simulink model "uavModel"  (R2023b)
settings: Solver=VariableStepAuto  StartTime=0.0  StopTime=10.0  RelTol=1e-3
InitFcn:
  | run('./config/config.m')
values from neighbouring files (symbols this model uses):
  mass = 11    [config_model.m]
undefined symbols (not defined in the file or in its folder): Cd, Cm, Earth, fractalcoef, lambda, propsMatrix, referenceHeight, WGS84, windSpeedInertial
libraries: aerolibasang x3, simulink_extras x1, aerolibtransform2 x1, aerolibatmos2 x1, shared6dof x1, sharedutil x1, sensorgpslib x1, mspsensorlib x1
settings Model: Creator=Rafael Blanco  LastModifiedBy=Victor

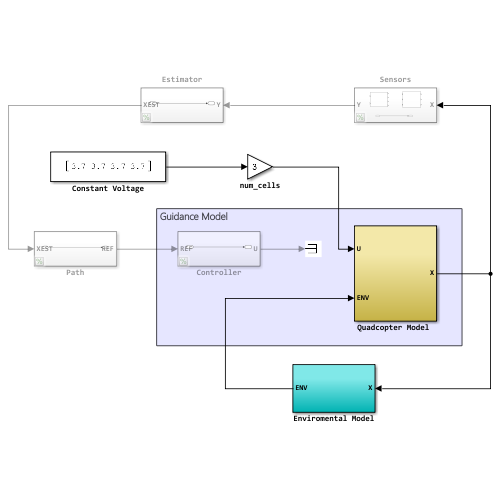
[thumbnail: Simulink's stored preview of the top-level diagram]
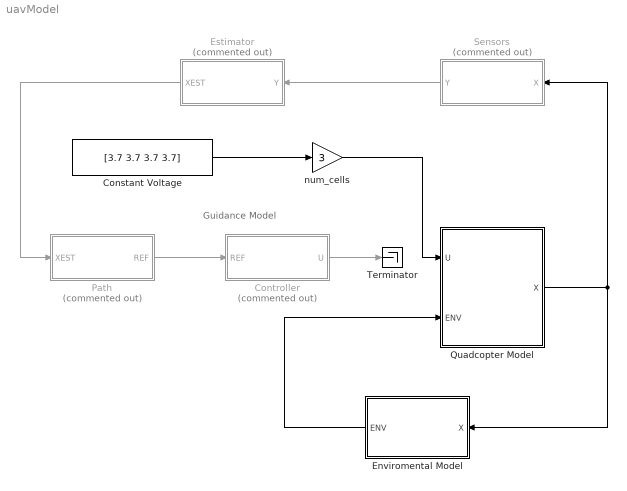
== system uavModel ==
  note: Guidance Model
  Constant Voltage : Constant  Value=[3.7 3.7 3.7 3.7]
  Controller : Subsystem  Commented=on
  Enviromental Model : Subsystem
  Estimator : Subsystem  Commented=on
  Path : Subsystem  Commented=on
  "Quadcopter Model " : Subsystem
  Sensors : Subsystem  Commented=on
  Terminator : Terminator
  num_cells : Gain  Gain=3
  wires:
  "Quadcopter Model "/1(X) -> Enviromental Model/1(X), Sensors/1(X)
  Enviromental Model/1(ENV) -> "Quadcopter Model "/2(ENV)
  Sensors/1(Y) -> Estimator/1(Y)
  Estimator/1(XEST) -> Path/1(XEST)
  Path/1(REF) -> Controller/1(REF)
  Controller/1(U) -> Terminator/1
  Constant Voltage/1 -> num_cells/1
  num_cells/1 -> "Quadcopter Model "/1(U)

== system uavModel/Controller ==
  REF : Inport
  U : Outport
  wires:
  REF/1 -> U/1

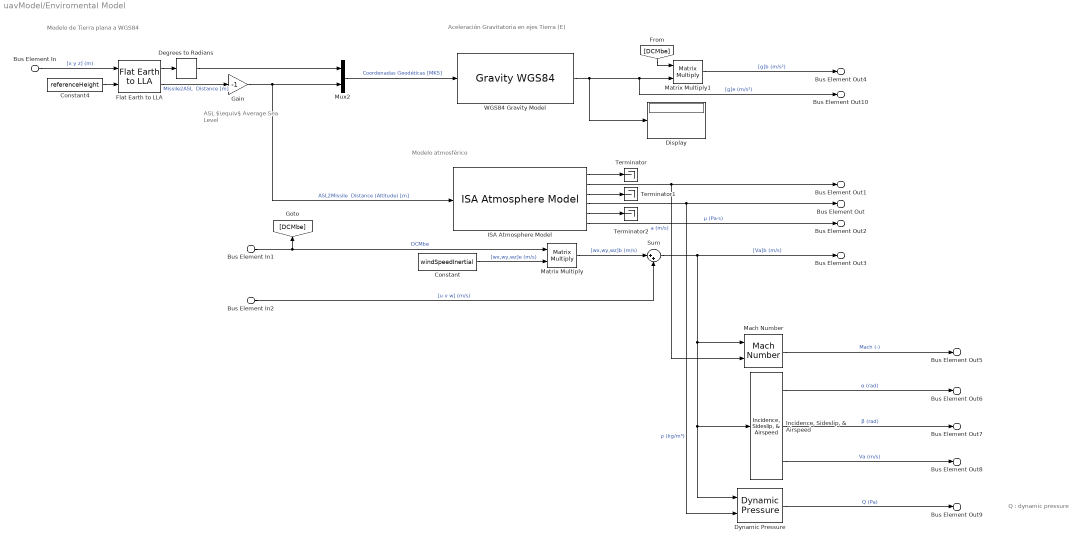
== system uavModel/Enviromental Model ==
  note: Modelo atmosférico
  note: Aceleración Gravitatoria en ejes Tierra (E)
  note: Modelo de Tierra plana a WGS84
  note: ASL $\equiv$ Average Sea Level
  note: Q : dynamic pressure
  Bus Element In2 : Inport  PortName=X  Element=[u v w] (m/s)
  Bus Element In : Inport  PortName=X  Element=[x y z] (m)
  Bus Element In1 : Inport  PortName=X  Element=DCMbe
  Constant : Constant  Value=windSpeedInertial
  Constant4 : Constant  Value=referenceHeight
  Degrees to Radians : simulink_extras/Transformations/Degrees to Radians
  Display : Display
  Dynamic Pressure : aerolibasang/Dynamic Pressure
  Flat Earth to LLA : aerolibtransform2/Flat Earth to LLA  units=Metric (MKS)  ptype=Earth (WGS84)  F=1/298.257223563  R=6378137  refPosPort=off  LL0=referenceGeodeticPosition  psi=0
  Gain : Gain  Gain=-1
  ISA Atmosphere Model : aerolibatmos2/ISA Atmosphere Model  useExtended=off  action=Warning  custom=off  viscosityOut=on  g=9.80665  gamma=1.4  R=287.0531  L=0.0065  h_trop=11000  h_strat=20000  rho0=1.225  P0=101325  T0=288.15  h0=0
  "Incidence, Sideslip, & Airspeed" : aerolibasang/Incidence, Sideslip, & Airspeed
  Mach Number : aerolibasang/Mach Number
  Matrix Multiply : Product  Multiplication=Matrix(*)
  Matrix Multiply1 : Product  Multiplication=Matrix(*)
  Mux2 : Mux  Inputs=2
  Sum : Sum  Inputs=|++
  Terminator : Terminator
  Terminator1 : Terminator
  Terminator2 : Terminator
  "WGS84 Gravity Model  " : GravityWGS84
  Bus Element Out : Outport  PortName=ENV  Element=ρ (kg/m³)
  Bus Element Out1 : Outport  PortName=ENV  Element=a (m/s)
  Bus Element Out2 : Outport  PortName=ENV  Element=μ (Pa·s)
  Bus Element Out3 : Outport  PortName=ENV  Element=[Va]b (m/s)
  Bus Element Out4 : Outport  PortName=ENV  Element=[g]b (m/s²)
  Bus Element Out5 : Outport  PortName=ENV  Element=Mach (-)
  Bus Element Out6 : Outport  PortName=ENV  Element=α (rad)
  Bus Element Out7 : Outport  PortName=ENV  Element=β (rad)
  Bus Element Out8 : Outport  PortName=ENV  Element=Va (m/s)
  Bus Element Out9 : Outport  PortName=ENV  Element=Q (Pa)
  Bus Element Out10 : Outport  PortName=ENV  Element=[g]e (m/s²)
  wires:
  "WGS84 Gravity Model  "/1 -> Bus Element Out10/1, Matrix Multiply1/2, Display/1  "[g]e (m/s²)"
  Mux2/1 -> "WGS84 Gravity Model  "/1  "Coordenadas Geodéticas [MKS]"
  Gain/1 -> Mux2/2, ISA Atmosphere Model/1  "ASL2Missile  Distance (Altitude) [m]"
  Flat Earth to LLA/1 -> Degrees to Radians/1
  Degrees to Radians/1 -> Mux2/1
  Flat Earth to LLA/2 -> Gain/1  "Missile2ASL  Distance [m]"
  Constant4/1 -> Flat Earth to LLA/2
  Bus Element In/1 -> Flat Earth to LLA/1  "[x y z] (m)"
  ISA Atmosphere Model/1 -> Terminator/1
  ISA Atmosphere Model/3 -> Terminator1/1
  ISA Atmosphere Model/4 -> Dynamic Pressure/2, Bus Element Out/1  "ρ (kg/m³)"
  Constant/1 -> Matrix Multiply/2  "[wx,wy,wz]e (m/s)"
  Matrix Multiply/1 -> Sum/1  "[wx,wy,wz]b (m/s)"
  Sum/1 -> Bus Element Out3/1, Mach Number/1, Dynamic Pressure/1, "Incidence, Sideslip, & Airspeed"/1  "[Va]b (m/s)"
  Bus Element In1/1 -> Matrix Multiply/1, [DCMbe]  "DCMbe"
  Matrix Multiply1/1 -> Bus Element Out4/1  "[g]b (m/s²)"
  [DCMbe] -> Matrix Multiply1/1
  ISA Atmosphere Model/5 -> Terminator2/1
  ISA Atmosphere Model/6 -> Bus Element Out2/1  "μ (Pa·s)"
  "Incidence, Sideslip, & Airspeed"/3 -> Bus Element Out8/1  "Va (m/s)"
  ISA Atmosphere Model/2 -> Mach Number/2, Bus Element Out1/1  "a (m/s)"
  Bus Element In2/1 -> Sum/2  "[u v w] (m/s)"
  Mach Number/1 -> Bus Element Out5/1  "Mach (-)"
  "Incidence, Sideslip, & Airspeed"/1 -> Bus Element Out6/1  "α (rad)"
  "Incidence, Sideslip, & Airspeed"/2 -> Bus Element Out7/1  "β (rad)"
  Dynamic Pressure/1 -> Bus Element Out9/1  "Q (Pa)"

== system uavModel/Estimator ==
  Y : Inport
  XEST : Outport
  wires:
  Y/1 -> XEST/1

== system uavModel/Path ==
  XEST : Inport
  REF : Outport
  wires:
  XEST/1 -> REF/1

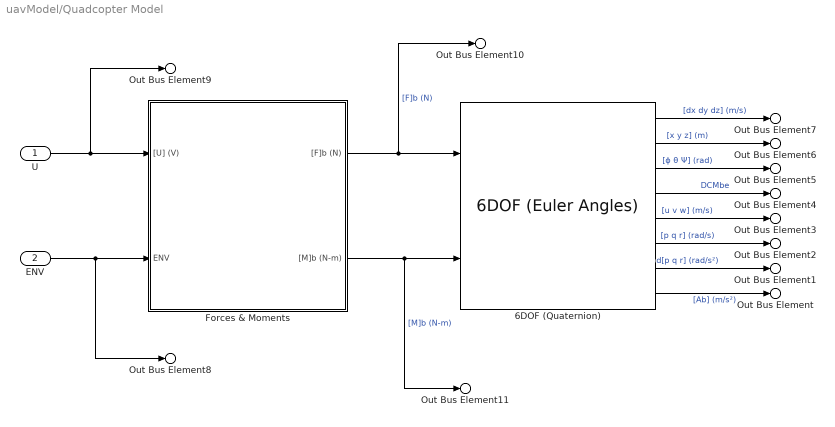
== system uavModel/Quadcopter Model  ==
  U : Inport
  ENV : Inport  Port=2
  6DOF (Quaternion) : shared6dof/6DOF (Euler Angles)  units=Metric (MKS)  mtype=Fixed  rep=Euler Angles  xme_0=initialPositionInertial  Vm_0=initialVelocityBody  eul_0=initialEulerAngles  pm_0=initialRatesBody  mass_0=mass  mass_e=0.5  mass_f=2.0  inertia=I  inertia_e=eye(3)  inertia_f=2*eye(3)  k_quat=1.0  vre_flag=on  abi_flag=off  aMode=aMode  xme_statename=''  Vm_statename=''  eul_statename=''  quat_statename=''  pm_statename=''  mass_statename=''
  Forces & Moments : Subsystem
  Out Bus Element : Outport  PortName=X  Element=[Ab] (m/s²)
  Out Bus Element1 : Outport  PortName=X  Element=d[p q r] (rad/s²)
  Out Bus Element2 : Outport  PortName=X  Element=[p q r] (rad/s)
  Out Bus Element3 : Outport  PortName=X  Element=[u v w] (m/s)
  Out Bus Element4 : Outport  PortName=X  Element=DCMbe
  Out Bus Element5 : Outport  PortName=X  Element=[ϕ θ Ψ] (rad)
  Out Bus Element6 : Outport  PortName=X  Element=[x y z] (m)
  Out Bus Element7 : Outport  PortName=X  Element=[dx dy dz] (m/s)
  Out Bus Element8 : Outport  PortName=X  Element=ENV
  Out Bus Element9 : Outport  PortName=X  Element=U
  Out Bus Element10 : Outport  PortName=X  Element=[F]b (N)
  Out Bus Element11 : Outport  PortName=X  Element=[M]b (N-m)
  wires:
  6DOF (Quaternion)/7 -> Out Bus Element1/1  "d[p q r] (rad/s²)"
  6DOF (Quaternion)/8 -> Out Bus Element/1  "[Ab] (m/s²)"
  6DOF (Quaternion)/6 -> Out Bus Element2/1  "[p q r] (rad/s)"
  6DOF (Quaternion)/5 -> Out Bus Element3/1  "[u v w] (m/s)"
  6DOF (Quaternion)/4 -> Out Bus Element4/1  "DCMbe"
  6DOF (Quaternion)/3 -> Out Bus Element5/1  "[ϕ θ Ψ] (rad)"
  6DOF (Quaternion)/2 -> Out Bus Element6/1  "[x y z] (m)"
  6DOF (Quaternion)/1 -> Out Bus Element7/1  "[dx dy dz] (m/s)"
  U/1 -> Forces & Moments/1("[U] (V)"), Out Bus Element9/1
  ENV/1 -> Forces & Moments/2(ENV), Out Bus Element8/1
  Forces & Moments/2("[M]b (N-m)") -> 6DOF (Quaternion)/2, Out Bus Element11/1  "[M]b (N-m)"
  Forces & Moments/1("[F]b (N)") -> 6DOF (Quaternion)/1, Out Bus Element10/1  "[F]b (N)"

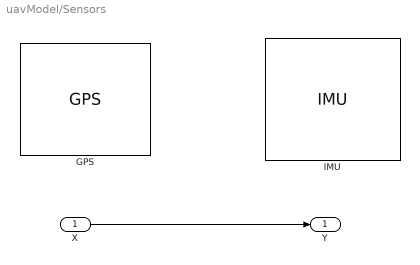
== system uavModel/Sensors ==
  X : Inport
  GPS : sensorgpslib/GPS  DispRefFrame=NED  PositionInputFormat=Local  ReferenceLocation=[ 0, 0, 0 ]  HorizontalPositionAccuracy=1.6  VerticalPositionAccuracy=3  VelocityAccuracy=0.1  DecayFactor=0.999  SeedDouble=67  SimulateUsing=Interpreted execution
      settings: LibrarySourceBlock=mspsensorlib/GPS
  IMU : mspsensorlib/IMU  DispRefFrame=NED  TemperaturePort=off  Temperature=25  MagneticFieldPort=off  MagneticFieldNED=[ 27.5550, -2.4169, -16.0849 ]  MagneticFieldENU=[ -2.4169, 27.5550, 16.0849 ]  SeedDouble=67  SimulateUsing=Interpreted execution  AccelParamsMeasurementRange=Inf  AccelParamsResolution=0  AccelParamsConstantBias=[ 0, 0, 0 ]  AccelParamsAxesMisalignment=[ 100, 0, 0; 0, 100, 0; 0, 0, 100 ]  AccelParamsNoiseDensity=[ 0, 0, 0 ]  AccelParamsBiasInstability=[ 0, 0, 0 ]  AccelParamsBiasInstabilityNumerator=fractalcoef().Numerator  AccelParamsBiasInstabilityDenominator=fractalcoef().Denominator  AccelParamsRandomWalk=[ 0, 0, 0 ]  AccelParamsNoiseType=double-sided  AccelParamsTemperatureBias=[ 0, 0, 0 ]  AccelParamsTemperatureScaleFactor=[ 0, 0, 0 ]  GyroParamsMeasurementRange=Inf  GyroParamsResolution=0  GyroParamsConstantBias=[ 0, 0, 0 ]  GyroParamsAxesMisalignment=[ 100, 0, 0; 0, 100, 0; 0, 0, 100 ]  GyroParamsAccelerationBias=[ 0, 0, 0 ]  GyroParamsNoiseDensity=[ 0, 0, 0 ]  GyroParamsBiasInstability=[ 0, 0, 0 ]  GyroParamsBiasInstabilityNumerator=fractalcoef().Numerator  GyroParamsBiasInstabilityDenominator=fractalcoef().Denominator  GyroParamsRandomWalk=[ 0, 0, 0 ]  GyroParamsNoiseType=double-sided  GyroParamsTemperatureBias=[ 0, 0, 0 ]  GyroParamsTemperatureScaleFactor=[ 0, 0, 0 ]  MagParamsMeasurementRange=Inf  MagParamsResolution=0  MagParamsConstantBias=[ 0, 0, 0 ]  MagParamsAxesMisalignment=[ 100, 0, 0; 0, 100, 0; 0, 0, 100 ]  MagParamsNoiseDensity=[ 0, 0, 0 ]  MagParamsBiasInstability=[ 0, 0, 0 ]  MagParamsBiasInstabilityNumerator=fractalcoef().Numerator  MagParamsBiasInstabilityDenominator=fractalcoef().Denominator  MagParamsRandomWalk=[ 0, 0, 0 ]  MagParamsNoiseType=double-sided  MagParamsTemperatureBias=[ 0, 0, 0 ]  MagParamsTemperatureScaleFactor=[ 0, 0, 0 ]
  Y : Outport
  wires:
  X/1 -> Y/1

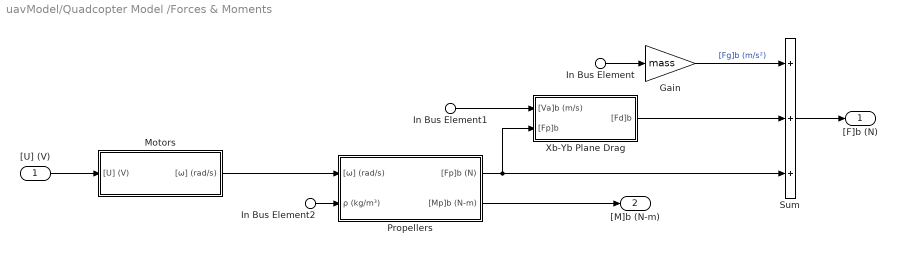
== system uavModel/Quadcopter Model /Forces & Moments ==
  "[U] (V)" : Inport
  In Bus Element : Inport  Port=2  PortName=ENV  Element=[g]b (m/s²)
  In Bus Element1 : Inport  Port=2  PortName=ENV  Element=[Va]b (m/s)
  In Bus Element2 : Inport  Port=2  PortName=ENV  Element=ρ (kg/m³)
  Gain : Gain  Gain=mass
  Motors : Subsystem
  Propellers : Subsystem
  Sum : Sum  Inputs=+++
  Xb-Yb Plane Drag : Subsystem
  "[F]b (N)" : Outport
  "[M]b (N-m)" : Outport  Port=2
  wires:
  "[U] (V)"/1 -> Motors/1("[U] (V)")
  Gain/1 -> Sum/1  "[Fg]b (m/s²)"
  Xb-Yb Plane Drag/1("[Fd]b") -> Sum/2
  Propellers/1("[Fp]b (N)") -> Xb-Yb Plane Drag/2("[Fp]b"), Sum/3
  In Bus Element/1 -> Gain/1
  Propellers/2("[Mp]b (N-m)") -> "[M]b (N-m)"/1
  In Bus Element1/1 -> Xb-Yb Plane Drag/1("[Va]b (m/s)")
  Sum/1 -> "[F]b (N)"/1
  In Bus Element2/1 -> Propellers/2(ρ (kg/m³))
  Motors/1("[ω] (rad/s)") -> Propellers/1("[ω] (rad/s)")

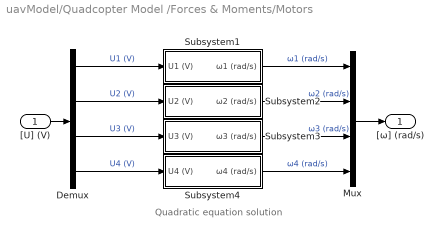
== system uavModel/Quadcopter Model /Forces & Moments/Motors ==
  note: Quadratic equation solution
  "[U] (V)" : Inport
  Demux : Demux
  Mux : Mux
  Subsystem1 : Subsystem
  Subsystem2 : Subsystem
  Subsystem3 : Subsystem
  Subsystem4 : Subsystem
  "[ω] (rad/s)" : Outport
  wires:
  "[U] (V)"/1 -> Demux/1
  Demux/1 -> Subsystem1/1(U1 (V))  "U1 (V)"
  Demux/2 -> Subsystem2/1(U2 (V))  "U2 (V)"
  Demux/3 -> Subsystem3/1(U3 (V))  "U3 (V)"
  Demux/4 -> Subsystem4/1(U4 (V))  "U4 (V)"
  Subsystem1/1(ω1 (rad/s)) -> Mux/1  "ω1 (rad/s)"
  Subsystem2/1(ω2 (rad/s)) -> Mux/2  "ω2 (rad/s)"
  Subsystem3/1(ω3 (rad/s)) -> Mux/3  "ω3 (rad/s)"
  Subsystem4/1(ω4 (rad/s)) -> Mux/4  "ω4 (rad/s)"
  Mux/1 -> "[ω] (rad/s)"/1

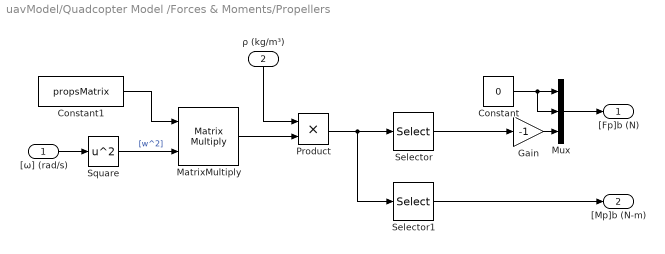
== system uavModel/Quadcopter Model /Forces & Moments/Propellers ==
  "[ω] (rad/s)" : Inport
  ρ (kg/m³) : Inport  Port=2
  Constant : Constant  Value=0
  Constant1 : Constant  Value=propsMatrix
  Gain : Gain  Gain=-1
  MatrixMultiply : Product  Multiplication=Matrix(*)
  Mux : Mux  Inputs=3
  Product : Product
  Selector : Selector  InputPortWidth=4  IndexOptions=Index vector (dialog)  Indices=[1]  OutputSizes=1
  Selector1 : Selector  InputPortWidth=4  IndexOptions=Index vector (dialog)  Indices=[2 3 4]  OutputSizes=1
  Square : Math  Operator=square
  "[Fp]b (N)" : Outport
  "[Mp]b (N-m)" : Outport  Port=2
  wires:
  "[ω] (rad/s)"/1 -> Square/1
  Mux/1 -> "[Fp]b (N)"/1
  Gain/1 -> Mux/3
  Constant/1 -> Mux/2, Mux/1
  Selector/1 -> Gain/1
  Selector1/1 -> "[Mp]b (N-m)"/1
  MatrixMultiply/1 -> Product/2
  Product/1 -> Selector1/1, Selector/1
  ρ (kg/m³)/1 -> Product/1
  Constant1/1 -> MatrixMultiply/1
  Square/1 -> MatrixMultiply/2  "[w^2]"

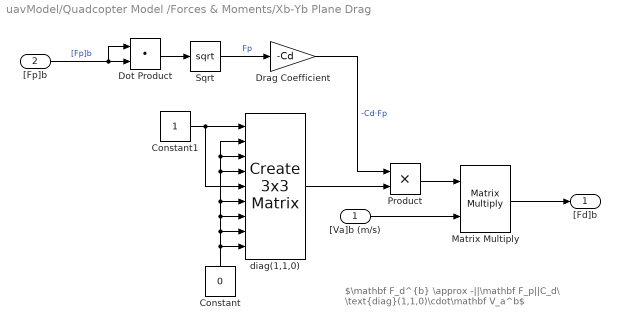
== system uavModel/Quadcopter Model /Forces & Moments/Xb-Yb Plane Drag ==
  note: $\mathbf F_d^{b} \approx -||\mathbf F_p||C_d\ \text{diag}(1,1,0)\cdot\mathbf V_a^b$
  "[Va]b (m/s)" : Inport
  "[Fp]b" : Inport  Port=2
  Constant : Constant  Value=0
  Constant1 : Constant
  Dot Product : DotProduct  OutDataTypeStr=Inherit: Inherit via internal rule
  Drag Coefficient : Gain  Gain=-Cd
  Matrix Multiply : Product  Multiplication=Matrix(*)
  Product : Product
  Sqrt : Sqrt
  diag(1,1,0) : sharedutil/Create 3x3 Matrix  aMode=aMode
      settings: LibrarySourceBlock=aerolibutil/Create 3x3 Matrix
  "[Fd]b" : Outport
  wires:
  "[Va]b (m/s)"/1 -> Matrix Multiply/2
  Constant/1 -> diag(1,1,0)/8, diag(1,1,0)/7, diag(1,1,0)/6, diag(1,1,0)/4, diag(1,1,0)/2, diag(1,1,0)/3, diag(1,1,0)/9
  diag(1,1,0)/1 -> Product/2
  Matrix Multiply/1 -> "[Fd]b"/1
  Sqrt/1 -> Drag Coefficient/1  "Fp"
  Drag Coefficient/1 -> Product/1  "-Cd·Fp"
  Dot Product/1 -> Sqrt/1
  "[Fp]b"/1 -> Dot Product/1, Dot Product/2  "[Fp]b"
  Product/1 -> Matrix Multiply/1
  Constant1/1 -> diag(1,1,0)/5, diag(1,1,0)/1

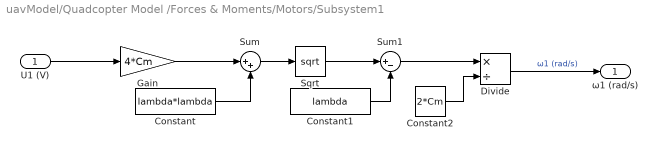
== system uavModel/Quadcopter Model /Forces & Moments/Motors/Subsystem1 ==
  U1 (V) : Inport
  Constant : Constant  Value=lambda*lambda
  Constant1 : Constant  Value=lambda
  Constant2 : Constant  Value=2*Cm
  Divide : Product  Inputs=*/
  Gain : Gain  Gain=4*Cm
  Sqrt : Sqrt
  Sum : Sum  Inputs=|++
  Sum1 : Sum  Inputs=|+-
  ω1 (rad/s) : Outport
  wires:
  Constant1/1 -> Sum1/2
  U1 (V)/1 -> Gain/1
  Sqrt/1 -> Sum1/1
  Constant2/1 -> Divide/2
  Constant/1 -> Sum/2
  Sum1/1 -> Divide/1
  Sum/1 -> Sqrt/1
  Gain/1 -> Sum/1
  Divide/1 -> ω1 (rad/s)/1  "ω1 (rad/s)"

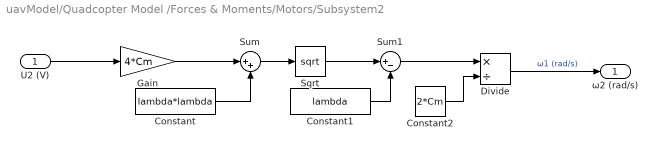
== system uavModel/Quadcopter Model /Forces & Moments/Motors/Subsystem2 ==
  U2 (V) : Inport
  Constant : Constant  Value=lambda*lambda
  Constant1 : Constant  Value=lambda
  Constant2 : Constant  Value=2*Cm
  Divide : Product  Inputs=*/
  Gain : Gain  Gain=4*Cm
  Sqrt : Sqrt
  Sum : Sum  Inputs=|++
  Sum1 : Sum  Inputs=|+-
  ω2 (rad/s) : Outport
  wires:
  Constant1/1 -> Sum1/2
  U2 (V)/1 -> Gain/1
  Sqrt/1 -> Sum1/1
  Constant2/1 -> Divide/2
  Constant/1 -> Sum/2
  Sum1/1 -> Divide/1
  Sum/1 -> Sqrt/1
  Gain/1 -> Sum/1
  Divide/1 -> ω2 (rad/s)/1  "ω1 (rad/s)"

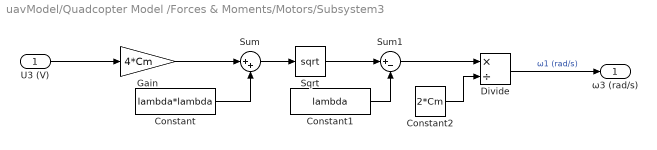
== system uavModel/Quadcopter Model /Forces & Moments/Motors/Subsystem3 ==
  U3 (V) : Inport
  Constant : Constant  Value=lambda*lambda
  Constant1 : Constant  Value=lambda
  Constant2 : Constant  Value=2*Cm
  Divide : Product  Inputs=*/
  Gain : Gain  Gain=4*Cm
  Sqrt : Sqrt
  Sum : Sum  Inputs=|++
  Sum1 : Sum  Inputs=|+-
  ω3 (rad/s) : Outport
  wires:
  Constant1/1 -> Sum1/2
  U3 (V)/1 -> Gain/1
  Sqrt/1 -> Sum1/1
  Constant2/1 -> Divide/2
  Constant/1 -> Sum/2
  Sum1/1 -> Divide/1
  Sum/1 -> Sqrt/1
  Gain/1 -> Sum/1
  Divide/1 -> ω3 (rad/s)/1  "ω1 (rad/s)"

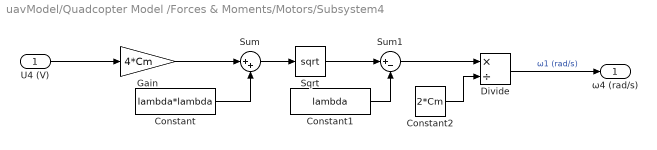
== system uavModel/Quadcopter Model /Forces & Moments/Motors/Subsystem4 ==
  U4 (V) : Inport
  Constant : Constant  Value=lambda*lambda
  Constant1 : Constant  Value=lambda
  Constant2 : Constant  Value=2*Cm
  Divide : Product  Inputs=*/
  Gain : Gain  Gain=4*Cm
  Sqrt : Sqrt
  Sum : Sum  Inputs=|++
  Sum1 : Sum  Inputs=|+-
  ω4 (rad/s) : Outport
  wires:
  Constant1/1 -> Sum1/2
  U4 (V)/1 -> Gain/1
  Sqrt/1 -> Sum1/1
  Constant2/1 -> Divide/2
  Constant/1 -> Sum/2
  Sum1/1 -> Divide/1
  Sum/1 -> Sqrt/1
  Gain/1 -> Sum/1
  Divide/1 -> ω4 (rad/s)/1  "ω1 (rad/s)"
